simulink model "d"  (R2020a)
settings: Solver=FixedStepAuto  StartTime=0  StopTime=10.67  FixedStep=0.01  RelTol=1e-3
undefined symbols (not defined in the file): delay, PSM, VSM
settings Model: Creator=yizha  LastModifiedBy=Brock
settings DataIOCC: ReturnWorkspaceOutputs=off
settings DebuggingCC: ArithmeticOperatorsInVariantConditions=warning
settings SFSimCC: CustomCodeUndefinedFunction=UseInterfaceOnly

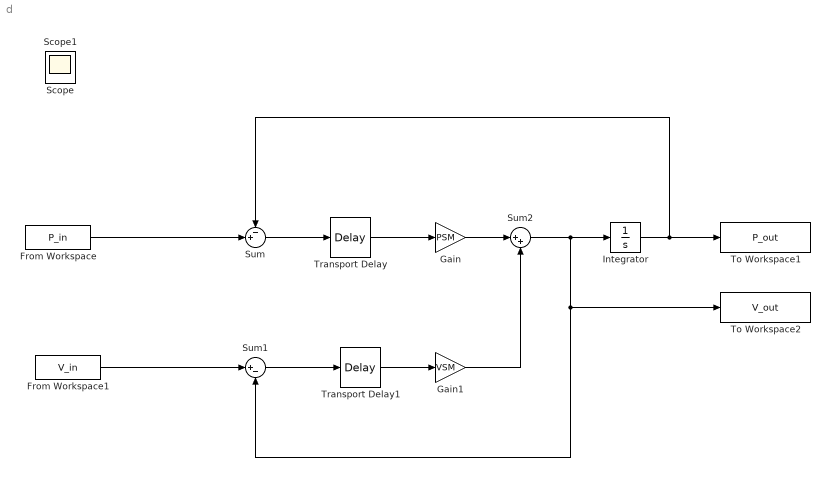
== system d ==
  From Workspace : FromWorkspace  VariableName=P_in
  From Workspace1 : FromWorkspace  VariableName=V_in
  Gain : Gain  Gain=PSM
  Gain1 : Gain  Gain=VSM
  Integrator : Integrator
  Sum : Sum  Inputs=-+|
  Sum1 : Sum  Inputs=|+-
  Sum2 : Sum  Inputs=|++
  To Workspace1 : ToWorkspace  VariableName=P_out  SampleTime=-1
  To Workspace2 : ToWorkspace  VariableName=V_out  SampleTime=-1
  Transport Delay : TransportDelay  DelayTime=delay
  Transport Delay1 : TransportDelay  DelayTime=delay
  Scope : Scope
  Scope1 : Scope
  wires:
  Sum/1 -> Transport Delay/1
  Transport Delay/1 -> Gain/1
  Integrator/1 -> To Workspace1/1, Sum/1
  From Workspace1/1 -> Sum1/1
  Sum1/1 -> Transport Delay1/1
  Transport Delay1/1 -> Gain1/1
  Gain/1 -> Sum2/1
  Sum2/1 -> Integrator/1, Sum1/2, To Workspace2/1
  Gain1/1 -> Sum2/2
  From Workspace/1 -> Sum/2
